simulink library "PowerElectronicsHandler"  (R2016b)
settings: Solver=VariableStepAuto  StartTime=0.0  StopTime=10.0  RelTol=1e-3
settings Model: Creator=Nathan  LastModifiedBy=march

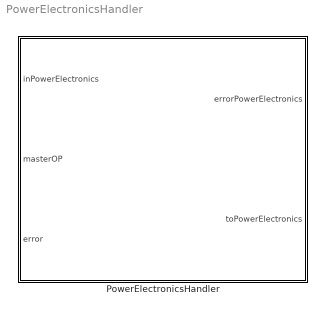
== system PowerElectronicsHandler ==
  PowerElectronicsHandler : Subsystem

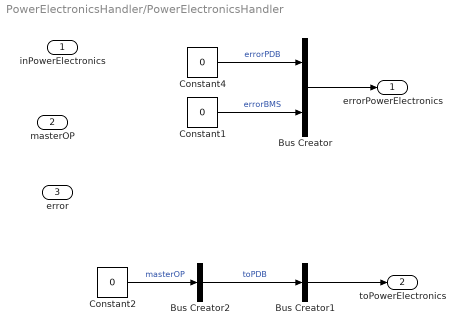
== system PowerElectronicsHandler/PowerElectronicsHandler ==
  inPowerElectronics : Inport  OutDataTypeStr=Bus: inPowerElectronics  BusOutputAsStruct=on
  masterOP : Inport  Port=2
  error : Inport  Port=3
  Bus Creator : BusCreator  Inputs=2
  Bus Creator1 : BusCreator  Inputs=1  OutDataTypeStr=Bus: toPowerElectronics
  Bus Creator2 : BusCreator  Inputs=1  OutDataTypeStr=Bus: toPDB
  Constant1 : Constant  Value=0
      settings: OpenFcn=|
      | b = get_param(gcb,'value');
      | if (strcmp(b,'72')),
      |   set_param (gcb,'value','0');
      | else
      |   set_param(gcb,'value','72');
      | end;
  Constant2 : Constant  Value=0
      settings: OpenFcn=|
      | b = get_param(gcb,'value');
      | if (strcmp(b,'1')),
      |   set_param (gcb,'value','0');
      | else
      |   set_param(gcb,'value','1');
      | end;
  Constant4 : Constant  Value=0
      settings: OpenFcn=|
      | b = get_param(gcb,'value');
      | if (strcmp(b,'72')),
      |   set_param (gcb,'value','0');
      | else
      |   set_param(gcb,'value','72');
      | end;
  errorPowerElectronics : Outport  OutDataTypeStr=Bus: errorPowerElectronics
  toPowerElectronics : Outport  Port=2  OutDataTypeStr=Bus: toPowerElectronics
  wires:
  Bus Creator2/1 -> Bus Creator1/1  "toPDB"
  Bus Creator1/1 -> toPowerElectronics/1
  Constant2/1 -> Bus Creator2/1  "masterOP"
  Bus Creator/1 -> errorPowerElectronics/1
  Constant4/1 -> Bus Creator/1  "errorPDB"
  Constant1/1 -> Bus Creator/2  "errorBMS"
